simulink model "detect_ver2"  (R2016a)
settings: Solver=VariableStepAuto  StartTime=0.0  StopTime=1  RelTol=1e-3
undefined symbols (not defined in the file): fspecial, Rec, SDTV
libraries: visionconversions x3, visionanalysis x1, visionsources x1
settings Model: Creator=Yewly  LastModifiedBy=Yewly
settings GRTTargetCC: GeneratePreprocessorConditionals=Use local settings

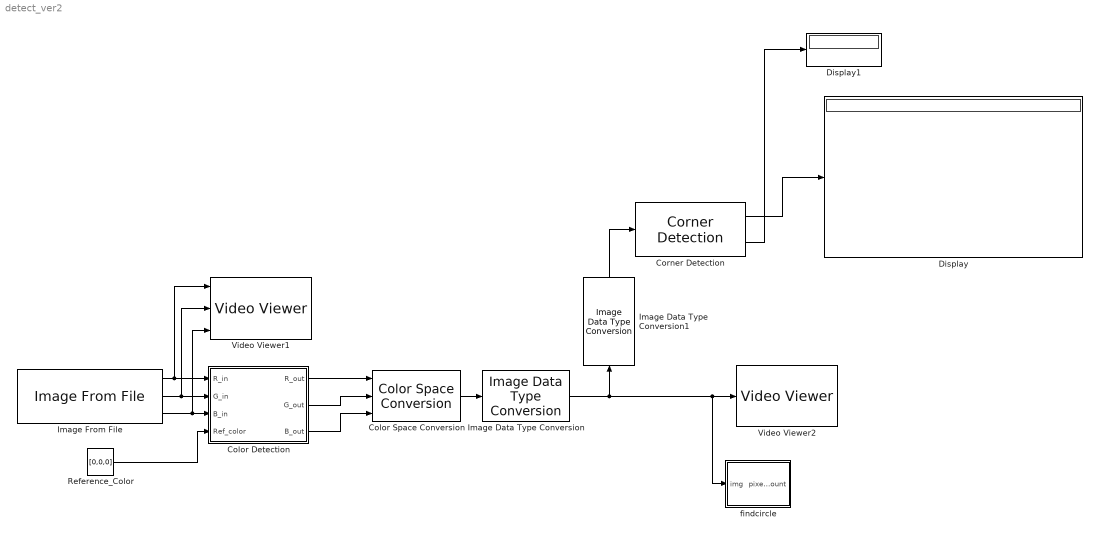
== system detect_ver2 ==
  Color Detection : Subsystem
  Color Space Conversion : visionconversions/Color Space  Conversion  conversion=Obsolete  conversionActive=R'G'B' to intensity  wp_str=D65  rec=Rec. 601 (SDTV)  sys=1125/60/2:1  imagePorts=Separate color signals
  Corner Detection : visionanalysis/Corner Detection  method=Harris corner detection (Harris & Stephens)  factor=0.04  filter=fspecial('gaussian', [1 5], 1.5)  thrInten=0.1  thrAngle=157.5  output=Obsolete9b  outputInUse=Corner location  maxNum=1000  thrMetric=0.005  neighborSize=[13 13]  isOutVarDim=off  accumMode=Binary point scaling  accumWordLength=32  accumFracLength=0  prodOutputMode=Binary point scaling  prodOutputWordLength=32  prodOutputFracLength=0  memoryMode=Binary point scaling  memoryWordLength=32  memoryFracLength=0  firstCoeffMode=Specify word length  firstCoeffWordLength=16  firstCoeffFracLength=16  roundingMode=Floor  overflowMode=off
  Display : Display
      settings: Decimation=100
  Display1 : Display
      settings: Decimation=100
  Image Data Type Conversion : visionconversions/Image Data Type Conversion  outDT=boolean  isSigned=on  wordLen=16  numFracBits=0
  Image Data Type Conversion1 : visionconversions/Image Data Type Conversion  outDT=double  isSigned=on  wordLen=16  numFracBits=0
  Image From File : visionsources/Image From File  Tag=vipblks_nd  FileName=color6.jpg  imagePorts=Separate color signals  Ts=1  ImageDataType=Inherit from input image  Signed=on  WordLength=16  sdImageDataType=uint(8)  FractionLengthMode=User-defined  FractionLength=15  OutPortLabels=R|G|B
  Reference_Color : Constant  Value=[0,0,0]  OutDataTypeStr=uint8
  Video Viewer1 : VideoViewer  imagePorts=separate color signals  FigPos=[380.2 748.4 540 585.6]
  Video Viewer2 : VideoViewer  FigPos=[133.8 735.6 540 585.6]
  "findcircle " : MATLAB Function  TreatAsAtomicUnit=on
  wires:
  Reference_Color/1 -> Color Detection/4(Ref_color)
  Color Detection/1(R_out) -> Color Space Conversion/1
  Image From File/1 -> Video Viewer1/1, Color Detection/1(R_in)
  Image From File/2 -> Video Viewer1/2, Color Detection/2(G_in)
  Image From File/3 -> Video Viewer1/3, Color Detection/3(B_in)
  Color Detection/2(G_out) -> Color Space Conversion/2
  Color Detection/3(B_out) -> Color Space Conversion/3
  Color Space Conversion/1 -> Image Data Type Conversion/1
  Image Data Type Conversion/1 -> Image Data Type Conversion1/1, "findcircle "/1(img), Video Viewer2/1
  Corner Detection/1 -> Display/1
  Corner Detection/2 -> Display1/1
  Image Data Type Conversion1/1 -> Corner Detection/1

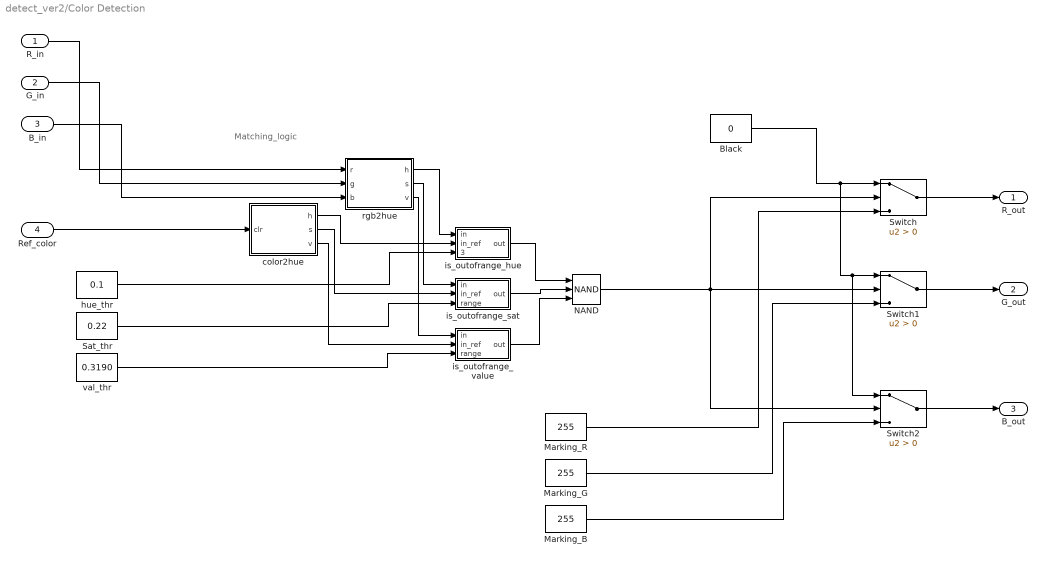
== system detect_ver2/Color Detection ==
  note: Matching_logic
  R_in : Inport
  G_in : Inport  Port=2
  B_in : Inport  Port=3
  Ref_color : Inport  Port=4
  Black : Constant  Value=0
  Marking_B : Constant  Value=255
  Marking_G : Constant  Value=255
  Marking_R : Constant  Value=255
  NAND : Logic  Operator=NAND  Inputs=3  IconShape=distinctive  AllPortsSameDT=off  OutDataTypeStr=boolean
  Sat_thr : Constant  Value=0.22
  Switch : Switch  Criteria=u2 > Threshold  OutDataTypeStr=uint8
  Switch1 : Switch  Criteria=u2 > Threshold  OutDataTypeStr=uint8
  Switch2 : Switch  Criteria=u2 > Threshold  OutDataTypeStr=uint8
  color2hue : MATLAB Function  TreatAsAtomicUnit=on
  hue_thr : Constant  Value=0.1
  is_outofrange_hue : Subsystem
  "is_outofrange_sat " : Subsystem
  is_outofrange_value : Subsystem
  rgb2hue : MATLAB Function  TreatAsAtomicUnit=on
  val_thr : Constant  Value=0.3190
  R_out : Outport
  G_out : Outport  Port=2
  B_out : Outport  Port=3
  wires:
  hue_thr/1 -> is_outofrange_hue/3("threshold ")
  is_outofrange_value/1(out) -> NAND/3
  is_outofrange_hue/1(out) -> NAND/1
  Sat_thr/1 -> "is_outofrange_sat "/3("range ")
  val_thr/1 -> is_outofrange_value/3("range ")
  rgb2hue/3(v) -> is_outofrange_value/1(in)
  color2hue/3(v) -> is_outofrange_value/2(in_ref)
  color2hue/1(h) -> is_outofrange_hue/2(in_ref)
  rgb2hue/1(h) -> is_outofrange_hue/1(in)
  Ref_color/1 -> color2hue/1(clr)
  "is_outofrange_sat "/1(out) -> NAND/2
  color2hue/2(s) -> "is_outofrange_sat "/2(in_ref)
  G_in/1 -> rgb2hue/2(g)
  rgb2hue/2(s) -> "is_outofrange_sat "/1(in)
  B_in/1 -> rgb2hue/3(b)
  R_in/1 -> rgb2hue/1(r)
  Marking_R/1 -> Switch/3
  Switch/1 -> R_out/1
  Switch1/1 -> G_out/1
  Switch2/1 -> B_out/1
  Marking_G/1 -> Switch1/3
  Marking_B/1 -> Switch2/3
  NAND/1 -> Switch2/2, Switch1/2, Switch/2
  Black/1 -> Switch2/1, Switch1/1, Switch/1

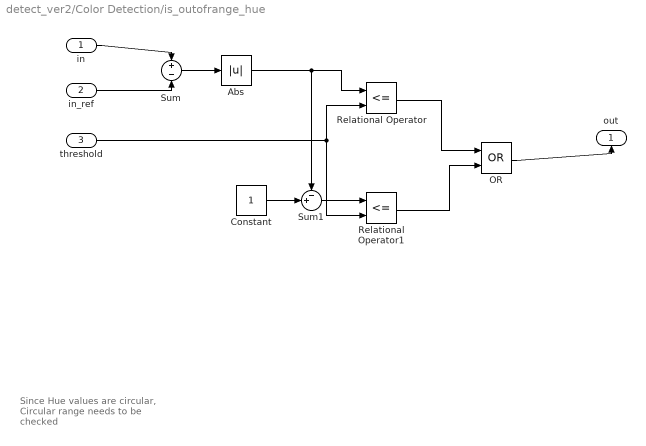
== system detect_ver2/Color Detection/is_outofrange_hue ==
  note: Since Hue values are circular, Circular range needs to be checked
  in : Inport
  in_ref : Inport  Port=2
  "threshold " : Inport  Port=3
  Abs : Abs
  Constant : Constant
  "OR " : Logic  Operator=OR  AllPortsSameDT=off  OutDataTypeStr=boolean
  Relational Operator : RelationalOperator  Operator=<=  OutDataTypeStr=boolean
  Relational Operator1 : RelationalOperator  Operator=<=  OutDataTypeStr=boolean
  Sum : Sum  Inputs=+|-
  Sum1 : Sum  Inputs=-+|
  out : Outport
  wires:
  in/1 -> Sum/1
  in_ref/1 -> Sum/2
  Sum/1 -> Abs/1
  Abs/1 -> Sum1/1, Relational Operator/1
  "threshold "/1 -> Relational Operator1/2, Relational Operator/2
  Constant/1 -> Sum1/2
  Sum1/1 -> Relational Operator1/1
  Relational Operator/1 -> "OR "/1
  Relational Operator1/1 -> "OR "/2
  "OR "/1 -> out/1

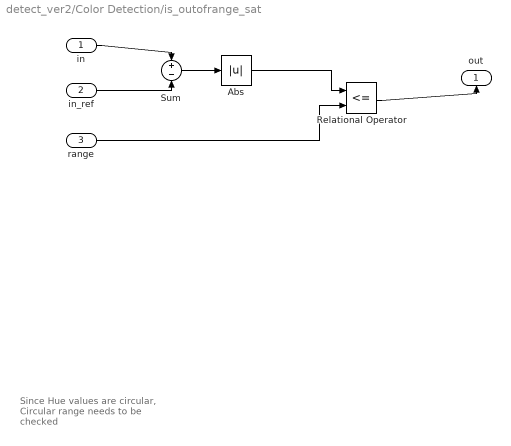
== system detect_ver2/Color Detection/is_outofrange_sat  ==
  note: Since Hue values are circular, Circular range needs to be checked
  in : Inport
  in_ref : Inport  Port=2
  "range " : Inport  Port=3
  Abs : Abs
  Relational Operator : RelationalOperator  Operator=<=  OutDataTypeStr=boolean
  Sum : Sum  Inputs=+|-
  out : Outport
  wires:
  in/1 -> Sum/1
  in_ref/1 -> Sum/2
  Sum/1 -> Abs/1
  Abs/1 -> Relational Operator/1
  "range "/1 -> Relational Operator/2
  Relational Operator/1 -> out/1

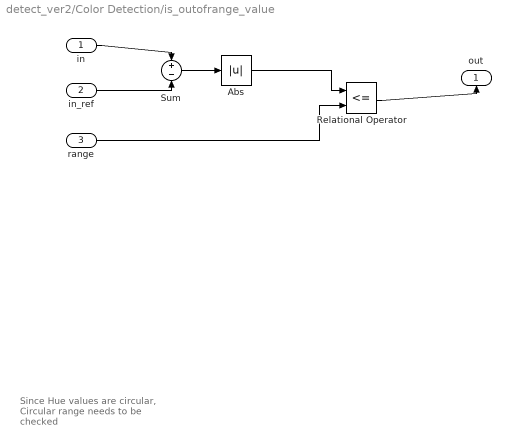
== system detect_ver2/Color Detection/is_outofrange_value ==
  note: Since Hue values are circular, Circular range needs to be checked
  in : Inport
  in_ref : Inport  Port=2
  "range " : Inport  Port=3
  Abs : Abs
  Relational Operator : RelationalOperator  Operator=<=  OutDataTypeStr=boolean
  Sum : Sum  Inputs=+|-
  out : Outport
  wires:
  in/1 -> Sum/1
  in_ref/1 -> Sum/2
  Sum/1 -> Abs/1
  Abs/1 -> Relational Operator/1
  "range "/1 -> Relational Operator/2
  Relational Operator/1 -> out/1

== matlab function detect_ver2/Color Detection/rgb2hue ==
  data: r input; h output; g input; b input; s output; v output
function [h,s,v] = rgb2hue(r,g,b)
%#codegen

sz = size(r);
r_re = double(reshape(r,[sz(1)*sz(2),1]))/255.0;
g_re = double(reshape(g,[sz(1)*sz(2),1]))/255.0;
b_re = double(reshape(b,[sz(1)*sz(2),1]))/255.0;
hsv = rgb2hsv([r_re,g_re,b_re]);
h = reshape(hsv(:,1), sz);
s = reshape(hsv(:,2), sz);
v = reshape(hsv(:,3), sz);

== matlab function detect_ver2/Color Detection/color2hue ==
  data: clr input; h output; s output; v output
function [h,s,v] = color2hue(clr)
%#codegen

hsv = rgb2hsv(double(clr')/255.0);
h = hsv(1);
s = hsv(2);
v = hsv(3);

== matlab function detect_ver2/findcircle  ==
  data: img input; pixel_count output
function pixel_count  = findcirle(img)
%#codegen
[h,w]= size(img);
pixel_count = sum(sum(img));
